simulink library "sys"  (R2021b)
settings: Solver=VariableStepAuto  StartTime=0.0  StopTime=10.0  RelTol=1e-3
undefined symbols (not defined in the file or in its folder): ENUM_NMMCURRENTSTATE_SLEEP, ENUM_PWRSTASW_OFF, ENUM_SYSNMMSTA_READYSLEEP, KSYS_SleepTimeBuffer_sec, TRUE, ZERO_FLOAT
libraries: simulink x4, hcu_lib x2
settings Model: Creator=Shawn  LastModifiedBy=FVT22063
settings SolverCC: AlgebraicLoopSolver=TrustRegion
settings DebuggingCC: SFMachineParentedDataDiag=warning

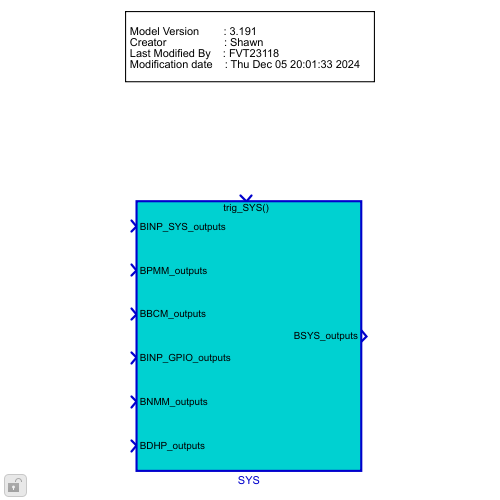
[thumbnail: Simulink's stored preview of the top-level diagram]
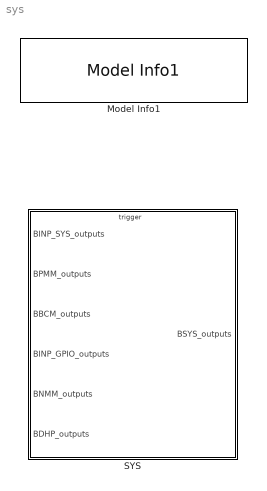
== system sys ==
  Model Info1 : hcu_lib/Model Info1  BlockCM=None  Frame=on  DisplayStringWithTags=|  HorizontalTextAlignment=Left  LeftAlignmentValue=0.02  SourceBlockDiagram=hcu_lib  TagMaxNumber=20
      | Model Version        : %<ModelVersion>
      | Creator                   : %<Creator>
      | Last Modified By    : %<LastModifiedBy>
      | Modification date    : %<LastModificationDate>
      settings: SourceProductName=HCU Relative Block Library
  SYS : Subsystem  TreatAsAtomicUnit=on
      settings: RTWSystemCode=Nonreusable function  RTWFcnNameOpts=Use subsystem name  RTWFileNameOpts=Use subsystem name

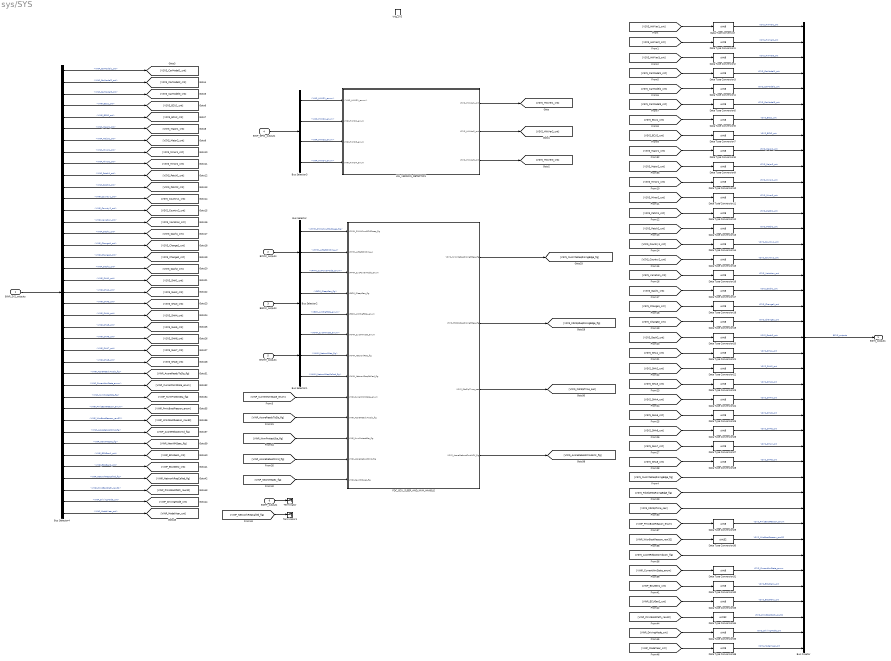
== system sys/SYS ==
  BINP_SYS_outputs : Inport  OutDataTypeStr=Bus: BINP_SYS_outputs
  BPMM_outputs : Inport  Port=2  OutDataTypeStr=Bus: BPMM_outputs
  BBCM_outputs : Inport  Port=3  OutDataTypeStr=Bus: BBCM_outputs
  BINP_GPIO_outputs : Inport  Port=4  OutDataTypeStr=Bus: BINP_GPIO_outputs
  BNMM_outputs : Inport  Port=5  OutDataTypeStr=Bus: BNMM_outputs
  BDHP_outputs : Inport  Port=6  OutDataTypeStr=Bus: BDHP_outputs
  trig_SYS : TriggerPort  TriggerType=function-call  VariantControl=(inherit)
  Bus Creator : BusCreator  Inputs=41  OutDataTypeStr=Bus: BSYS_outputs  NonVirtualBus=on
  Bus Selector : BusSelector  OutputSignals=VPMM_PMMAllowECUSleep_flg,VPMM_LVBattChktime_s,VPMM_SysPowerMode_enum
  Bus Selector1 : BusSelector  OutputSignals=VNMM_SysNMmSta_enum,VNMM_NetworkReq_flg,VNMM_NetworkReqCalled_flg
  Bus Selector2 : BusSelector  OutputSignals=VBCM_SleepReq_flg,VBCM_AntitheftSta_enum
  Bus Selector3 : BusSelector  OutputSignals=VINP_HWID1_enum,VINP_HWID2_enum,VINP_HWID3_enum,VINP_HWID4_enum
  Bus Selector4 : BusSelector  OutputSignals=VINP_CarModel1_cnt,VINP_CarModel2_cnt,VINP_CarModel3_cnt,VINP_ECU1_cnt,VINP_ECU2_cnt,VINP_Major1_cnt,VINP_Major2_cnt,VINP_Minor1_cnt,VINP_Minor2_cnt,VINP_Patch1_cnt,VINP_Patch2_cnt,VINP_Country1_cnt,VINP_Country2_cnt,VINP_Variation_cnt,VINP_Dash1_cnt,VINP_Change1_cnt,VINP_Change2_cnt,VINP_Dash2_cnt,VINP_SHA1_cnt,VINP_SHA2_cnt,VINP_SHA3_cnt,VINP_SHA4_cnt,VINP_SHA5_cnt,VINP_SHA6_cnt,VINP_SHA7_cnt,VINP_SHA8_cnt,VINP_AcoreReadyToSlp_flg,VINP_CurrentNmState_enum,VINP_NvmProtectSta_flg,VINP_PmicBootReason_enum,VINP_WisrBootReason_raw32,VINP_AcoreRebootCmd_flg,VINP_NewNMSpec_flg,VINP_ECUGen1_cnt,VINP_ECUGen2_cnt,VINP_NetworkReqCalled_flg,VINP_PmicBootPath_raw32,VINP_DrivingMode_cnt,VINP_ModelYear_cnt
  Data Type Conversion{,1..29,31..33,35..36} (35 alike) : DataTypeConversion  OutDataTypeStr=uint8
  Data Type Conversion30 : DataTypeConversion  OutDataTypeStr=uint32
  Data Type Conversion34 : DataTypeConversion  OutDataTypeStr=uint32
  FDC_ECU_SLEEP_AND_NVM_HANDLE : Subsystem
  HW_VERSION_DETECTION : Subsystem
  Terminator : Terminator
  Terminator1 : Terminator
  BSYS_outputs : Outport  OutDataTypeStr=Bus: BSYS_outputs
  wires:
  BPMM_outputs/1 -> Bus Selector/1
  BBCM_outputs/1 -> Bus Selector2/1
  Bus Creator/1 -> BSYS_outputs/1  "BSYS_outputs"
  BINP_SYS_outputs/1 -> Bus Selector4/1
  Bus Selector4/22 -> [VSYS_SHA4_cnt]  "<VINP_SHA4_cnt>"
  Bus Selector4/8 -> [VSYS_Minor1_cnt]  "<VINP_Minor1_cnt>"
  Bus Selector4/25 -> [VSYS_SHA7_cnt]  "<VINP_SHA7_cnt>"
  Bus Selector4/15 -> [VSYS_Dash1_cnt]  "<VINP_Dash1_cnt>"
  Bus Selector4/16 -> [VSYS_Change1_cnt]  "<VINP_Change1_cnt>"
  Bus Selector4/19 -> [VSYS_SHA1_cnt]  "<VINP_SHA1_cnt>"
  Bus Selector4/17 -> [VSYS_Change2_cnt]  "<VINP_Change2_cnt>"
  Bus Selector4/26 -> [VSYS_SHA8_cnt]  "<VINP_SHA8_cnt>"
  Bus Selector4/18 -> [VSYS_Dash2_cnt]  "<VINP_Dash2_cnt>"
  Bus Selector4/24 -> [VSYS_SHA6_cnt]  "<VINP_SHA6_cnt>"
  Bus Selector4/20 -> [VSYS_SHA2_cnt]  "<VINP_SHA2_cnt>"
  Bus Selector4/13 -> [VSYS_Country2_cnt]  "<VINP_Country2_cnt>"
  Bus Selector4/1 -> [VSYS_CarModel1_cnt]  "<VINP_CarModel1_cnt>"
  Bus Selector4/14 -> [VSYS_Variation_cnt]  "<VINP_Variation_cnt>"
  Bus Selector4/7 -> [VSYS_Major2_cnt]  "<VINP_Major2_cnt>"
  Bus Selector4/11 -> [VSYS_Patch2_cnt]  "<VINP_Patch2_cnt>"
  Bus Selector4/2 -> [VSYS_CarModel2_cnt]  "<VINP_CarModel2_cnt>"
  Bus Selector4/4 -> [VSYS_ECU1_cnt]  "<VINP_ECU1_cnt>"
  Bus Selector4/23 -> [VSYS_SHA5_cnt]  "<VINP_SHA5_cnt>"
  Bus Selector4/5 -> [VSYS_ECU2_cnt]  "<VINP_ECU2_cnt>"
  Bus Selector4/10 -> [VSYS_Patch1_cnt]  "<VINP_Patch1_cnt>"
  Bus Selector4/21 -> [VSYS_SHA3_cnt]  "<VINP_SHA3_cnt>"
  Bus Selector4/6 -> [VSYS_Major1_cnt]  "<VINP_Major1_cnt>"
  Bus Selector4/3 -> [VSYS_CarModel3_cnt]  "<VINP_CarModel3_cnt>"
  Bus Selector4/12 -> [VSYS_Country1_cnt]  "<VINP_Country1_cnt>"
  Bus Selector4/9 -> [VSYS_Minor2_cnt]  "<VINP_Minor2_cnt>"
  Bus Selector/1 -> FDC_ECU_SLEEP_AND_NVM_HANDLE/1(VPMM_PMMAllowECUSleep_flg)  "<VPMM_PMMAllowECUSleep_flg>"
  Bus Selector/2 -> FDC_ECU_SLEEP_AND_NVM_HANDLE/2(VPMM_LVBattChktime_s)  "<VPMM_LVBattChktime_s>"
  Bus Selector2/1 -> FDC_ECU_SLEEP_AND_NVM_HANDLE/4(VBCM_SleepReq_flg)  "<VBCM_SleepReq_flg>"
  Bus Selector4/27 -> [VINP_AcoreReadyToSlp_flg]  "<VINP_AcoreReadyToSlp_flg>"
  [VINP_AcoreReadyToSlp_flg] -> FDC_ECU_SLEEP_AND_NVM_HANDLE/10(VINP_AcoreReadyToSlp_flg)
  Bus Selector4/28 -> [VINP_CurrentNmState_enum]  "<VINP_CurrentNmState_enum>"
  [VINP_CurrentNmState_enum] -> FDC_ECU_SLEEP_AND_NVM_HANDLE/9(VINP_CurrentNmState_enum)
  [VSYS_FdcSlpReqRisingEdge_flg] -> Bus Creator/31
  [VSYS_NvWriteReqRisingEdge_flg] -> Bus Creator/30
  [VSYS_FdcSlpTime_sec] -> Bus Creator/32
  Bus Selector2/2 -> FDC_ECU_SLEEP_AND_NVM_HANDLE/5(VBCM_AntitheftSta_enum)  "<VBCM_AntitheftSta_enum>"
  Bus Selector3/4 -> HW_VERSION_DETECTION/4(VINP_HWID4_enum)  "<VINP_HWID4_enum>"
  Bus Selector3/1 -> HW_VERSION_DETECTION/1(<VINP_HWID1_enum>)  "<VINP_HWID1_enum>"
  Bus Selector3/3 -> HW_VERSION_DETECTION/3(VINP_HWID3_enum)  "<VINP_HWID3_enum>"
  BINP_GPIO_outputs/1 -> Bus Selector3/1
  Bus Selector3/2 -> HW_VERSION_DETECTION/2(VINP_HWID2_enum)  "<VINP_HWID2_enum>"
  HW_VERSION_DETECTION/1(VSYS_HWVer1_cnt) -> [VSYS_HWVer1_cnt]
  HW_VERSION_DETECTION/3(VSYS_HWVer3_cnt) -> [VSYS_HWVer3_cnt]
  HW_VERSION_DETECTION/2(VSYS_HWVer2_cnt) -> [VSYS_HWVer2_cnt]
  [VSYS_SHA6_cnt] -> Data Type Conversion26/1
  [VSYS_HWVer2_cnt] -> Data Type Conversion1/1
  [VSYS_SHA1_cnt] -> Data Type Conversion21/1
  [VSYS_Dash2_cnt] -> Data Type Conversion20/1
  Data Type Conversion/1 -> Bus Creator/1  "VSYS_HWVer1_cnt"
  [VSYS_CarModel2_cnt] -> Data Type Conversion4/1
  [VSYS_SHA5_cnt] -> Data Type Conversion25/1
  [VSYS_Change2_cnt] -> Data Type Conversion19/1
  Data Type Conversion28/1 -> Bus Creator/29  "VSYS_SHA8_cnt"
  Data Type Conversion8/1 -> Bus Creator/9  "VSYS_Major1_cnt"
  [VSYS_SHA8_cnt] -> Data Type Conversion28/1
  [VSYS_SHA4_cnt] -> Data Type Conversion24/1
  Data Type Conversion24/1 -> Bus Creator/25  "VSYS_SHA4_cnt"
  [VSYS_Patch1_cnt] -> Data Type Conversion12/1
  [VSYS_Dash1_cnt] -> Data Type Conversion17/1
  [VSYS_CarModel3_cnt] -> Data Type Conversion5/1
  Data Type Conversion18/1 -> Bus Creator/19  "VSYS_Change1_cnt"
  [VSYS_CarModel1_cnt] -> Data Type Conversion3/1
  [VSYS_SHA7_cnt] -> Data Type Conversion27/1
  [VSYS_HWVer1_cnt] -> Data Type Conversion/1
  [VSYS_SHA2_cnt] -> Data Type Conversion22/1
  Data Type Conversion9/1 -> Bus Creator/10  "VSYS_Major2_cnt"
  Data Type Conversion17/1 -> Bus Creator/18  "VSYS_Dash1_cnt"
  Data Type Conversion1/1 -> Bus Creator/2  "VSYS_HWVer2_cnt"
  Data Type Conversion15/1 -> Bus Creator/16  "VSYS_Country2_cnt"
  Data Type Conversion27/1 -> Bus Creator/28  "VSYS_SHA7_cnt"
  Data Type Conversion14/1 -> Bus Creator/15  "VSYS_Country1_cnt"
  Data Type Conversion4/1 -> Bus Creator/5  "VSYS_CarModel2_cnt"
  Data Type Conversion16/1 -> Bus Creator/17  "VSYS_Variation_cnt"
  Data Type Conversion10/1 -> Bus Creator/11  "VSYS_Minor1_cnt"
  [VSYS_Minor2_cnt] -> Data Type Conversion11/1
  Data Type Conversion11/1 -> Bus Creator/12  "VSYS_Minor2_cnt"
  [VSYS_Minor1_cnt] -> Data Type Conversion10/1
  Data Type Conversion20/1 -> Bus Creator/21  "VSYS_Dash2_cnt"
  Data Type Conversion23/1 -> Bus Creator/24  "VSYS_SHA3_cnt"
  Data Type Conversion25/1 -> Bus Creator/26  "VSYS_SHA5_cnt"
  [VSYS_SHA3_cnt] -> Data Type Conversion23/1
  Data Type Conversion22/1 -> Bus Creator/23  "VSYS_SHA2_cnt"
  Data Type Conversion19/1 -> Bus Creator/20  "VSYS_Change2_cnt"
  Data Type Conversion7/1 -> Bus Creator/8  "VSYS_ECU2_cnt"
  Data Type Conversion6/1 -> Bus Creator/7  "VSYS_ECU1_cnt"
  [VSYS_ECU2_cnt] -> Data Type Conversion7/1
  [VSYS_Variation_cnt] -> Data Type Conversion16/1
  Data Type Conversion26/1 -> Bus Creator/27  "VSYS_SHA6_cnt"
  [VSYS_Country2_cnt] -> Data Type Conversion15/1
  [VSYS_Patch2_cnt] -> Data Type Conversion13/1
  Data Type Conversion13/1 -> Bus Creator/14  "VSYS_Patch2_cnt"
  Data Type Conversion21/1 -> Bus Creator/22  "VSYS_SHA1_cnt"
  [VSYS_HWVer3_cnt] -> Data Type Conversion2/1
  Data Type Conversion3/1 -> Bus Creator/4  "VSYS_CarModel1_cnt"
  [VSYS_Major2_cnt] -> Data Type Conversion9/1
  Data Type Conversion5/1 -> Bus Creator/6  "VSYS_CarModel3_cnt"
  [VSYS_Change1_cnt] -> Data Type Conversion18/1
  [VSYS_Major1_cnt] -> Data Type Conversion8/1
  [VSYS_Country1_cnt] -> Data Type Conversion14/1
  Data Type Conversion12/1 -> Bus Creator/13  "VSYS_Patch1_cnt"
  Data Type Conversion2/1 -> Bus Creator/3  "VSYS_HWVer3_cnt"
  [VSYS_ECU1_cnt] -> Data Type Conversion6/1
  Bus Selector4/29 -> [VINP_NvmProtectSta_flg]  "<VINP_NvmProtectSta_flg>"
  [VINP_NvmProtectSta_flg] -> FDC_ECU_SLEEP_AND_NVM_HANDLE/11(VINP_NvmProtectSta_flg)
  BNMM_outputs/1 -> Bus Selector1/1
  Bus Selector1/1 -> FDC_ECU_SLEEP_AND_NVM_HANDLE/6(VNMM_SysNMmSta_enum)  "<VNMM_SysNMmSta_enum>"
  Data Type Conversion29/1 -> Bus Creator/33  "VSYS_PmicBootReason_enum"
  Data Type Conversion30/1 -> Bus Creator/34  "VSYS_WisrBootReason_raw32"
  Bus Selector4/30 -> [VINP_PmicBootReason_enum]  "<VINP_PmicBootReason_enum>"
  Bus Selector4/31 -> [VINP_WisrBootReason_raw32]  "<VINP_WisrBootReason_raw32>"
  [VINP_PmicBootReason_enum] -> Data Type Conversion29/1
  [VINP_WisrBootReason_raw32] -> Data Type Conversion30/1
  Bus Selector/3 -> FDC_ECU_SLEEP_AND_NVM_HANDLE/3(VPMM_SysPowerMode_enum)  "<VPMM_SysPowerMode_enum>"
  Bus Selector4/32 -> [VINP_AcoreRebootCmd_flg]  "<VINP_AcoreRebootCmd_flg>"
  [VINP_AcoreRebootCmd_flg] -> FDC_ECU_SLEEP_AND_NVM_HANDLE/12(VINP_AcoreRebootCmd_flg)
  [VSYS_AcoreRebootCmdACK_flg] -> Bus Creator/35
  [VINP_CurrentNmState_enum] -> Data Type Conversion31/1
  Data Type Conversion31/1 -> Bus Creator/36  "VSYS_CurrentNmState_enum"
  Bus Selector4/33 -> [VINP_NewNMSpec_flg]  "<VINP_NewNMSpec_flg>"
  [VINP_NewNMSpec_flg] -> FDC_ECU_SLEEP_AND_NVM_HANDLE/13(VINP_NewNMSpec_flg)
  Bus Selector4/34 -> [VINP_ECUGen1_cnt]  "<VINP_ECUGen1_cnt>"
  Bus Selector4/35 -> [VINP_ECUGen2_cnt]  "<VINP_ECUGen2_cnt>"
  [VINP_ECUGen1_cnt] -> Data Type Conversion32/1
  [VINP_ECUGen2_cnt] -> Data Type Conversion33/1
  Data Type Conversion32/1 -> Bus Creator/37  "VSYS_ECUGen1_cnt"
  Data Type Conversion33/1 -> Bus Creator/38  "VSYS_ECUGen2_cnt"
  BDHP_outputs/1 -> Terminator/1
  Bus Selector4/36 -> [VINP_NetworkReqCalled_flg]  "<VINP_NetworkReqCalled_flg>"
  Bus Selector1/2 -> FDC_ECU_SLEEP_AND_NVM_HANDLE/7(VNMM_NetworkReq_flg)  "<VNMM_NetworkReq_flg>"
  Bus Selector4/37 -> [VINP_PmicBootPath_raw32]  "<VINP_PmicBootPath_raw32>"
  [VINP_PmicBootPath_raw32] -> Data Type Conversion34/1
  Data Type Conversion34/1 -> Bus Creator/39  "VSYS_PmicBootPath_raw32"
  [VINP_NetworkReqCalled_flg] -> Terminator1/1
  Bus Selector1/3 -> FDC_ECU_SLEEP_AND_NVM_HANDLE/8(VNMM_NetworkReqCalled_flg)  "<VNMM_NetworkReqCalled_flg>"
  Bus Selector4/38 -> [VINP_DrivingMode_cnt]  "<VINP_DrivingMode_cnt>"
  Bus Selector4/39 -> [VINP_ModelYear_cnt]  "<VINP_ModelYear_cnt>"
  [VINP_DrivingMode_cnt] -> Data Type Conversion35/1
  [VINP_ModelYear_cnt] -> Data Type Conversion36/1
  Data Type Conversion35/1 -> Bus Creator/40  "VSYS_DrivingMode_cnt"
  Data Type Conversion36/1 -> Bus Creator/41  "VSYS_ModelYear_cnt"
  FDC_ECU_SLEEP_AND_NVM_HANDLE/1(VSYS_NvWriteReqRisingEdge_flg) -> [VSYS_NvWriteReqRisingEdge_flg]
  FDC_ECU_SLEEP_AND_NVM_HANDLE/2(VSYS_FdcSlpReqRisingEdge_flg) -> [VSYS_FdcSlpReqRisingEdge_flg]
  FDC_ECU_SLEEP_AND_NVM_HANDLE/3(VSYS_FdcSlpTime_sec) -> [VSYS_FdcSlpTime_sec]
  FDC_ECU_SLEEP_AND_NVM_HANDLE/4(VSYS_AcoreRebootCmdACK_flg) -> [VSYS_AcoreRebootCmdACK_flg]

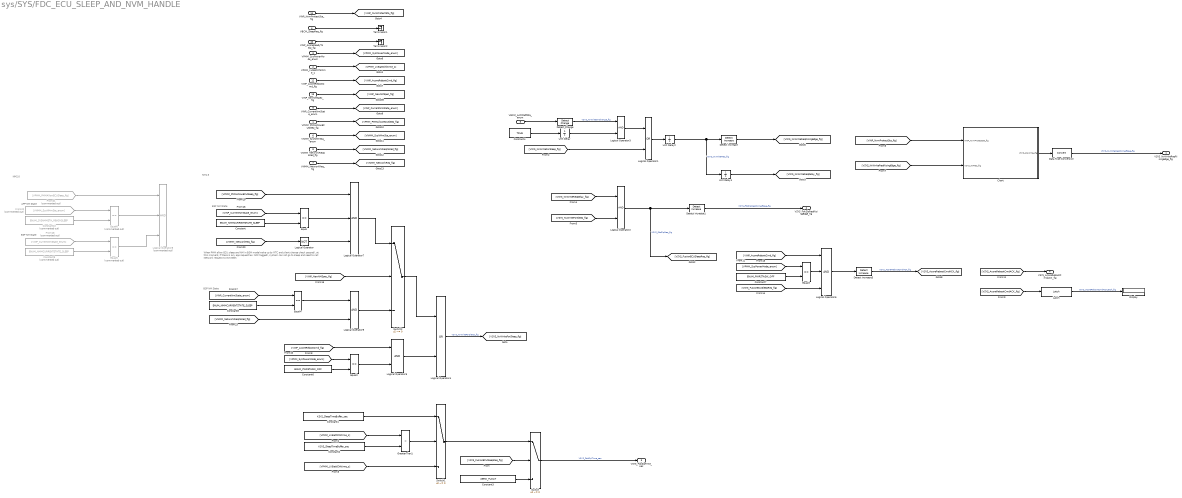
== system sys/SYS/FDC_ECU_SLEEP_AND_NVM_HANDLE ==
  note: When PMM allow ECU sleep and NM in BSM mode(wake up by RTC and silent charge check passed),
      | at this moment, if there is any app request(ex: NFC tagged),
      | system can not go to sleep and need to call Network request to exit BSM.
  note: NM1.5
  note: NM2.0
  note: BSP NM State
  note: BSP NM State
  note: APP NM State
  note: BSP NM State
  VPMM_PMMAllowECUSleep_flg : Inport
  VPMM_LVBattChktime_s : Inport  Port=2
  VPMM_SysPowerMode_enum : Inport  Port=3
  VBCM_SleepReq_flg : Inport  Port=4
  VBCM_AntitheftSta_enum : Inport  Port=5
  VNMM_SysNMmSta_enum : Inport  Port=6
  VNMM_NetworkReq_flg : Inport  Port=7
  VNMM_NetworkReqCalled_flg : Inport  Port=8
  VINP_CurrentNmState_enum : Inport  Port=9
  VINP_AcoreReadyToSlp_flg : Inport  Port=10
  VINP_NvmProtectSta_flg : Inport  Port=11
  VINP_AcoreRebootCmd_flg : Inport  Port=12
  VINP_NewNMSpec_flg : Inport  Port=13
  Chart : Stateflow chart  TreatAsAtomicUnit=on
  Constant : Constant  Value=ENUM_NMMCURRENTSTATE_SLEEP
  Constant1 : Constant  Value=KSYS_SleepTimeBuffer_sec
  Constant10 : Constant  Commented=on  Value=ENUM_SYSNMMSTA_READYSLEEP
  Constant2 : Constant  Value=KSYS_SleepTimeBuffer_sec
  Constant3 : Constant  Value=ZERO_FLOAT
  Constant4 : Constant  Value=TRUE
  Constant6 : Constant  Value=ENUM_PWRSTASW_OFF
  Constant7 : Constant  Value=ENUM_PWRSTASW_OFF
  Constant8 : Constant  Value=ENUM_NMMCURRENTSTATE_SLEEP
  Constant9 : Constant  Commented=on  Value=ENUM_NMMCURRENTSTATE_SLEEP
  Data Type Conversion : DataTypeConversion
  Detect Change : simulink/Logic and Bit Operations/Detect Change  vinit=0  OutDataTypeStr=boolean
  Detect Increase : simulink/Logic and Bit Operations/Detect Increase  vinit=0.0  OutDataTypeStr=boolean
  Detect Increase1 : simulink/Logic and Bit Operations/Detect Increase  vinit=0.0  OutDataTypeStr=boolean
  Detect Increase3 : simulink/Logic and Bit Operations/Detect Increase  vinit=0.0  OutDataTypeStr=boolean
  Display : Display
  Equal{,2..4} (4 alike) : RelationalOperator  Operator===  OutDataTypeStr=boolean  RndMeth=Simplest
  Equal5 : RelationalOperator  Commented=on  Operator===  OutDataTypeStr=boolean  RndMeth=Simplest
  Equal6 : RelationalOperator  Commented=on  Operator===  OutDataTypeStr=boolean  RndMeth=Simplest
  From18 : From  Commented=on  GotoTag=VINP_CurrentNmState_enum
  From21 : From  Commented=on  GotoTag=VPMM_PMMAllowECUSleep_flg
  From22 : From  Commented=on  GotoTag=VNMM_SysNMmSta_enum
  GreaterThan1 : RelationalOperator  Operator=<  OutDataTypeStr=boolean  RndMeth=Simplest
  Latch : hcu_lib/Basic_Blocks/Latch
  Logical Operator : Logic  Operator=NOT  AllPortsSameDT=off  OutDataTypeStr=boolean
  Logical Operator1 : Logic  Operator=OR  AllPortsSameDT=off  OutDataTypeStr=boolean
  Logical Operator{2..3,5,9} (4 alike) : Logic  AllPortsSameDT=off  OutDataTypeStr=boolean
  Logical Operator4 : Logic  Operator=OR  AllPortsSameDT=off  OutDataTypeStr=boolean
  Logical Operator6 : Logic  Inputs=3  AllPortsSameDT=off  OutDataTypeStr=boolean
  Logical Operator7 : Logic  Inputs=3  AllPortsSameDT=off  OutDataTypeStr=boolean
  Logical Operator8 : Logic  Commented=on  Inputs=3  AllPortsSameDT=off  OutDataTypeStr=boolean
  Switch : Switch  Criteria=u2 ~= 0
      settings: AttributesFormatString=%<Criteria>
  Switch1 : Switch  Criteria=u2 ~= 0
      settings: AttributesFormatString=%<Criteria>
  Switch2 : Switch  Criteria=u2 ~= 0
      settings: AttributesFormatString=%<Criteria>
  Terminator1 : Terminator
  Terminator2 : Terminator
  Unit Delay : UnitDelay  SampleTime=-1  HasFrameUpgradeWarning=on
  Unit Delay1 : UnitDelay  SampleTime=-1  HasFrameUpgradeWarning=on
  Unit Delay2 : UnitDelay  SampleTime=-1  HasFrameUpgradeWarning=on
  VSYS_NvWriteReqRisingEdge_flg : Outport
  VSYS_FdcSlpReqRisingEdge_flg : Outport  Port=2
  VSYS_FdcSlpTime_sec : Outport  Port=3
  VSYS_AcoreRebootCmdACK_flg : Outport  Port=4
  wires:
  Switch1/1 -> Switch/1
  [VSYS_FusionECUSleepReq_flg] -> Switch/2
  VPMM_LVBattChktime_s/1 -> [VPMM_LVBattChktime_s]
  Switch/1 -> VSYS_FdcSlpTime_sec/1  "VSYS_FdcSlpTime_sec"
  [VPMM_LVBattChktime_s] -> GreaterThan1/1
  Constant2/1 -> GreaterThan1/2
  Constant3/1 -> Switch/3
  GreaterThan1/1 -> Switch1/2
  [VPMM_LVBattChktime_s] -> Switch1/3
  Constant1/1 -> Switch1/1
  Constant/1 -> Equal/2
  VBCM_AntitheftSta_enum/1 -> Detect Change/1
  [VSYS_NvWriteForSleep_flg] -> Logical Operator1/2
  Unit Delay2/1 -> Detect Increase/1, Unit Delay1/1  "VSYS_NvWriteReq_flg"
  Unit Delay1/1 -> [VSYS_NvWriteReqDelay_flg]
  [VSYS_NvWriteReqDelay_flg] -> Logical Operator2/1
  [VSYS_NvWriteForSleep_flg] -> Logical Operator2/2
  Logical Operator2/1 -> Detect Increase1/1, [VSYS_FusionECUSleepReq_flg]  "VSYS_FdcSlpReq_flg"
  Detect Change/1 -> Logical Operator3/1  "VSYS_NvWriteOnChange_flg"
  Unit Delay/1 -> Logical Operator3/2
  Constant4/1 -> Unit Delay/1
  Logical Operator3/1 -> Logical Operator1/1
  Detect Increase1/1 -> VSYS_FdcSlpReqRisingEdge_flg/1  "VSYS_FdcSlpReqRisingEdge_flg"
  Logical Operator1/1 -> Unit Delay2/1
  VBCM_SleepReq_flg/1 -> Terminator1/1
  VINP_AcoreReadyToSlp_flg/1 -> Terminator2/1
  Detect Increase/1 -> [VSYS_NvWriteReqRisingEdge_flg]
  Chart/1(VSYS_DoWrite_flg) -> Data Type Conversion/1
  Data Type Conversion/1 -> VSYS_NvWriteReqRisingEdge_flg/1  "VSYS_NvWriteReqRisingEdge_flg"
  [VSYS_NvWriteReqRisingEdge_flg] -> Chart/2(VSYS_WrReq_flg)
  [VINP_NvmProtectSta_flg] -> Chart/1(VINP_NvmProtectSta_flg)
  VINP_NvmProtectSta_flg/1 -> [VINP_NvmProtectSta_flg]
  Logical Operator4/1 -> [VSYS_NvWriteForSleep_flg]  "VSYS_NvWriteForSleep_flg"
  Equal2/1 -> Logical Operator5/2
  Logical Operator5/1 -> Logical Operator4/2
  [VINP_AcoreRebootCmd_flg] -> Logical Operator5/1
  VPMM_SysPowerMode_enum/1 -> [VPMM_SysPowerMode_enum]
  [VPMM_SysPowerMode_enum] -> Equal2/1
  Constant6/1 -> Equal2/2
  VINP_AcoreRebootCmd_flg/1 -> [VINP_AcoreRebootCmd_flg]
  [VSYS_AcoreRebootCmdACK_flg] -> VSYS_AcoreRebootCmdACK_flg/1
  [VSYS_AcoreRebootCmdACK_flg] -> Latch/1
  Latch/1 -> Display/1  "VSYS_AcoreRebootCmdACKLatch_flg"
  Constant7/1 -> Equal3/2
  [VPMM_SysPowerMode_enum] -> Equal3/1
  [VINP_AcoreRebootCmd_flg] -> Logical Operator6/1
  Equal3/1 -> Logical Operator6/2
  Logical Operator6/1 -> Detect Increase3/1
  [VSYS_FusionECUSleepReq_flg] -> Logical Operator6/3
  Detect Increase3/1 -> [VSYS_AcoreRebootCmdACK_flg]  "VSYS_AcoreRebootCmdACK_flg"
  Equal/1 -> Logical Operator7/2
  VINP_NewNMSpec_flg/1 -> [VINP_NewNMSpec_flg]
  [VINP_NewNMSpec_flg] -> Switch2/2
  Logical Operator7/1 -> Switch2/1
  Switch2/1 -> Logical Operator4/1
  VINP_CurrentNmState_enum/1 -> [VINP_CurrentNmState_enum]
  [VINP_CurrentNmState_enum] -> Equal/1
  [VINP_CurrentNmState_enum] -> Equal4/1
  Constant8/1 -> Equal4/2
  Equal4/1 -> Logical Operator9/1
  Constant10/1 -> Equal6/2
  Equal5/1 -> Logical Operator8/3
  From18/1 -> Equal5/1
  From22/1 -> Equal6/1
  Constant9/1 -> Equal5/2
  From21/1 -> Logical Operator8/1
  Equal6/1 -> Logical Operator8/2
  VPMM_PMMAllowECUSleep_flg/1 -> [VPMM_PMMAllowECUSleep_flg]
  [VPMM_PMMAllowECUSleep_flg] -> Logical Operator7/1
  VNMM_SysNMmSta_enum/1 -> [VNMM_SysNMmSta_enum]
  [VNMM_NetworkReq_flg] -> Logical Operator/1
  Logical Operator/1 -> Logical Operator7/3
  VNMM_NetworkReqCalled_flg/1 -> [VNMM_NetworkReqCalled_flg]
  [VNMM_NetworkReqCalled_flg] -> Logical Operator9/2
  Logical Operator9/1 -> Switch2/3
  VNMM_NetworkReq_flg/1 -> [VNMM_NetworkReq_flg]

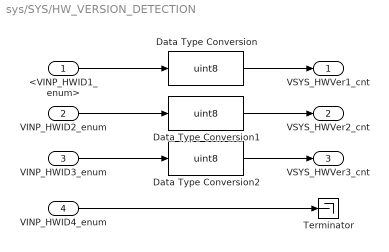
== system sys/SYS/HW_VERSION_DETECTION ==
  <VINP_HWID1_enum> : Inport
  VINP_HWID2_enum : Inport  Port=2
  VINP_HWID3_enum : Inport  Port=3
  VINP_HWID4_enum : Inport  Port=4
  Data Type Conversion : DataTypeConversion  OutDataTypeStr=uint8
  Data Type Conversion1 : DataTypeConversion  OutDataTypeStr=uint8
  Data Type Conversion2 : DataTypeConversion  OutDataTypeStr=uint8
  Terminator : Terminator
  VSYS_HWVer1_cnt : Outport
  VSYS_HWVer2_cnt : Outport  Port=2
  VSYS_HWVer3_cnt : Outport  Port=3
  wires:
  Data Type Conversion/1 -> VSYS_HWVer1_cnt/1
  Data Type Conversion1/1 -> VSYS_HWVer2_cnt/1
  VINP_HWID3_enum/1 -> Data Type Conversion2/1
  Data Type Conversion2/1 -> VSYS_HWVer3_cnt/1
  <VINP_HWID1_enum>/1 -> Data Type Conversion/1
  VINP_HWID2_enum/1 -> Data Type Conversion1/1
  VINP_HWID4_enum/1 -> Terminator/1

== stateflow chart sys/SYS/FDC_ECU_SLEEP_AND_NVM_HANDLE/Chart ==
  state NvmProtectJudge
    (default) -> (junction 30) : {
        |  VSYS_DoWriteMemory_flg = 0;
        |  VSYS_DoWrite_flg = 0;
        |  }
    NvmProtectJudge -> (junction 30)
    (junction 30) -> (junction 31) [order 1] : [VSYS_WrReq_flg || VSYS_DoWriteMemory_flg]
    (junction 31) -> (junction 35) [order 1] : [VINP_NvmProtectSta_flg]
    (junction 30) -> (junction 32) [order 2] : {VSYS_DoWrite_flg = 0;}
    (junction 31) -> (junction 38) [order 2] : {
        |  VSYS_DoWriteMemory_flg = 0;
        |  VSYS_DoWrite_flg = 1;
        |  }
    (junction 35) -> (junction 39) : {
        |  VSYS_DoWriteMemory_flg = 1;
        |  VSYS_DoWrite_flg = 0;
        |  }
    (junction 38) -> (junction 32)
    (junction 39) -> (junction 38)
  (default) -> NvmProtectJudge
  data: VINP_NvmProtectSta_flg input; VSYS_WrReq_flg input; VSYS_DoWrite_flg output; VSYS_DoWriteMemory_flg local boolean
